simulink model "input_test"  (R2017a)
settings: Solver=FixedStepAuto  StartTime=0.0  StopTime=500  FixedStep=0.1  RelTol=1e-3
undefined symbols (not defined in the file): sigbuilder_block
libraries: simulink x1
settings Model: Creator=Sidharth Agarwal  LastModifiedBy=Sidharth Agarwal

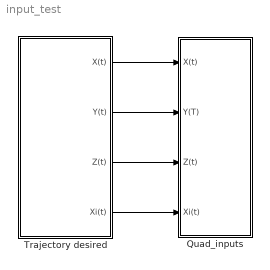
== system input_test ==
  Quad_inputs : Subsystem
  Trajectory desired : Subsystem
  wires:
  Trajectory desired/1(X(t)) -> Quad_inputs/1(X(t))
  Trajectory desired/2(Y(t)) -> Quad_inputs/2(Y(T))
  Trajectory desired/3(Z(t)) -> Quad_inputs/3(Z(t))
  Trajectory desired/4(Xi(t)) -> Quad_inputs/4(Xi(t))

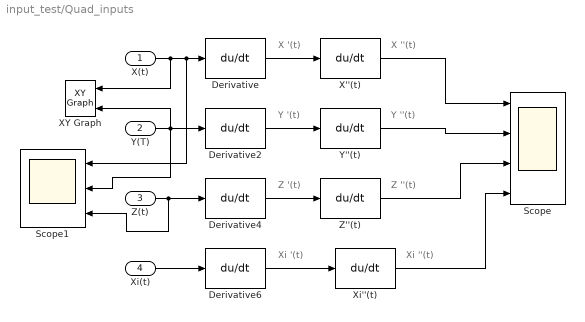
== system input_test/Quad_inputs ==
  note: Xi ''(t)
  note: X '(t)
  note: Y '(t)
  note: Z '(t)
  note: Xi '(t)
  note: X ''(t)
  note: Y ''(t)
  note: Z ''(t)
  X(t) : Inport
  Y(T) : Inport  Port=2
  Z(t) : Inport  Port=3
  Xi(t) : Inport  Port=4
  Derivative{,2,4,6} (4 alike) : Derivative
  Scope : Scope  NumInputPorts=4
  Scope1 : Scope  NumInputPorts=3
  X''(t) : Derivative
  XY Graph : simulink/Sinks/XY Graph  xmin=-5  xmax=20  ymin=-5  ymax=20  st=-1
  Xi''(t) : Derivative
  Y''(t) : Derivative
  Z''(t) : Derivative
  wires:
  X(t)/1 -> XY Graph/1, Scope1/1, Derivative/1
  Derivative/1 -> X''(t)/1
  Derivative2/1 -> Y''(t)/1
  Y(T)/1 -> Scope1/2, XY Graph/2, Derivative2/1
  Derivative4/1 -> Z''(t)/1
  Z(t)/1 -> Scope1/3, Derivative4/1
  Derivative6/1 -> Xi''(t)/1
  Xi(t)/1 -> Derivative6/1
  Xi''(t)/1 -> Scope/4
  X''(t)/1 -> Scope/1
  Y''(t)/1 -> Scope/2
  Z''(t)/1 -> Scope/3

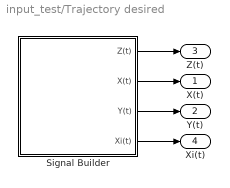
== system input_test/Trajectory desired ==
  Signal Builder : Subsystem  Tag=STV Subsys  LoadFcn=sigbuilder_block('load');  StartFcn=sigbuilder_block('start');  StopFcn=sigbuilder_block('stop');  ClipboardFcn=sigbuilder_block('clipboard');  mask(Sigbuilder block){tuvar=[0:10]}
      mask help: Simulink:masks:SigbuilderBlock_MD
      mask init:
      | if ~strcmp(get_param(bdroot(gcbh),'SimulationStatus'),'stopped') tuvar = sigbuilder_block('maskInit'); end
      settings: CopyFcn=sigbuilder_block('copy');  DeleteFcn=sigbuilder_block('delete');  ModelCloseFcn=sigbuilder_block('modelClose');  PreSaveFcn=sigbuilder_block('preSave');  PauseFcn=sigbuilder_block('pause');  ContinueFcn=sigbuilder_block('continue');  NameChangeFcn=sigbuilder_block('namechange');  OpenFcn=sigbuilder_block('open',[0 30 1024.5 488.25 ]);  CloseFcn=sigbuilder_block('close');
      mask Display: plot(0, 0, 100, 100,[2, 2, 32, 32, 2], [68, 8, 8, 68, 68],[32, 2], [38, 38], [32, 19, 2],[53, 60, 44], [32, 17, 17, 2],[16, 16, 31, 31]);txt = getActiveGroup(gcbh);text(2, 100, txt,'verticalAlignment', 'top');
  X(t) : Outport
  Y(t) : Outport  Port=2
  Z(t) : Outport  Port=3
  Xi(t) : Outport  Port=4
  wires:
  Signal Builder/1(Z(t)) -> Z(t)/1
  Signal Builder/2(X(t)) -> X(t)/1
  Signal Builder/3(Y(t)) -> Y(t)/1
  Signal Builder/4(Xi(t)) -> Xi(t)/1

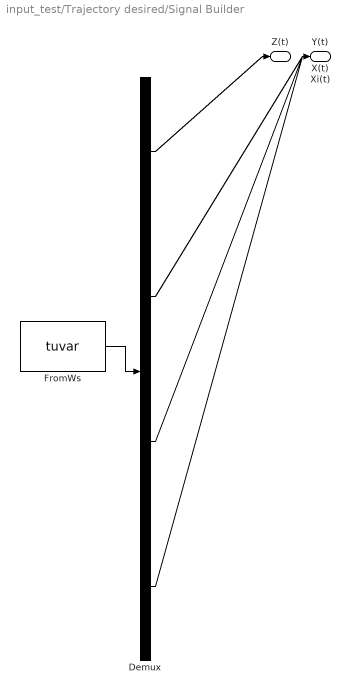
== system input_test/Trajectory desired/Signal Builder ==
  Demux : Demux  Tag=STV Demux
  FromWs : FromWorkspace  Tag=STV FromWs  VariableName=tuvar  SampleTime=0
      SigBuilderData=|
      | common.afterFinalStr = 'Extrapolate'
      | common.sampleTime = 0
      | dataSet.timeRange = [0 500]
      | dataSet.name = 'Pos(t)'
      | sbobj.Groups.Name = 'Pos(t)'
      | sbobj.Groups.Signals(1).Name = 'Z(t)'
      | sbobj.Groups.Signals(1).XData = [0 2 50 500]
      | sbobj.Groups.Signals(1).YData = [0 0.38 6 6]
      | sbobj.Groups.Signals(2).Name = 'X(t)'
      | sbobj.Groups.Signals(2).XData = [0 50 90 120 160 190 230 260 300 330 370 400 440 500]
      | sbobj.Groups.Signals(2).YData = [0 3 10 10 0 0 10 10 0 0 10 10 0 0]
      | sbobj.Groups.Signals(3).Name = 'Y(t)'
      | sbobj.Groups.Signals(3).XData = [0 90 120 160 190 230 260 300 330 370 400 500]
      | sbobj.Groups.Signals(3).YData = [0 0 3 3 6 6 9 9 12 12 15 15]
      | sbobj.Groups.Signals(4).Name = 'Xi(t)'
      | sbobj.Groups.Signals(4).XData = [0 500]
      | sbobj.Groups.Signals(4).YData = [0 0]
      | sbobj.Groups.TimeRange = [0 500]
  Z(t) : Outport  Tag=STV Outport
  X(t) : Outport  Tag=STV Outport  Port=2
  Y(t) : Outport  Tag=STV Outport  Port=3
  Xi(t) : Outport  Tag=STV Outport  Port=4
  wires:
  FromWs/1 -> Demux/1
  Demux/1 -> Z(t)/1
  Demux/2 -> X(t)/1
  Demux/3 -> Y(t)/1
  Demux/4 -> Xi(t)/1
